simulink model "entropyModel"  (R2024a)
settings: Solver=ode45  StartTime=0.0  StopTime=500  MaxStep=0.1  RelTol=1e-6  AbsTol=1e-6  EnableMultiTasking=on
PreLoadFcn:
  | entropyModelParam;
InitFcn:
  | entropyModelParam;
model workspace (MAT data in the model file):
  cBall = 1000
  cBorder = 1000
  tRegBall = 0.0001
  tRegBorder = 0.0001
undefined symbols (not defined in the file): S1, S10, S2, S3, S4, S5, S6, S7, S8, S9, squareDim, X, Y, Z
libraries: sm_lib x18, nesl_utility x1
settings Model: Creator=lnicolet  LastModifiedBy=lnicolet
settings SolverCC: AutoScaleAbsTol=off  AlgebraicLoopSolver=TrustRegion  MaxZcPerStep=1
settings DataIOCC: LimitDataPoints=on  MaxDataPoints=10000  SaveOutput=off  DSMLogging=off  SaveTime=off  ReturnWorkspaceOutputsName=entropyModelOut
settings OptimizationCC: ReuseModelBlockBuffer=off  LifeSpan=inf
settings DebuggingCC: UnconnectedInputMsg=warning  UnconnectedOutputMsg=warning  UnconnectedLineMsg=warning  AllowSymbolicDim=off  SubsystemReferenceDiagnosticForUnitTest=warning  SFUnexpectedBacktrackingDiag=warning  SFNoUnconditionalDefaultTransitionDiag=warning  SFExecutionAtInitializationDiag=none  ArithmeticOperatorsInVariantConditions=warning
settings ModelReferenceCC: EnableRefExpFcnMdlSchedulingChecks=on
settings SFSimCC: SimUseLocalCustomCode=off  CustomCodeUndefinedFunction=UseInterfaceOnly
settings RTWCC: RTWUseLocalCustomCode=off  GPUComputeCapability=3.5  DLArmComputeVersion=19.05
settings CodeAppCC: StateflowObjectComments=on
settings GRTTargetCC: TargetLangStandard=C89/C90 (ANSI)
settings ConfigComp: CovMetricSettings=dw  CovSaveCumulativeToWorkspaceVar=on  CovSaveSingleToWorkspaceVar=on  CovExternalEMLEnable=off  CovSFcnEnable=off
settings SimscapeCC: SimscapeLogType=all  SimscapeLogSimulationStatistics=on  SimscapeLogLimitData=off  SimscapeLogDataHistory=10000
settings ExplorerConfigSet: InternalSimMechanicsExplorerSettings="<ExplorerConfiguration><canonicalview>default</canonicalview><AnimationSetting><BasePlaybackSpeed>1.0</BasePlaybackSpeed><PlaybackSpeedFactor>8.0</PlaybackSpeedFactor></AnimationSetting><TilePanel><TileInfo><Tiles Columns=\"1\" Count=\"1\" Rows=\"1\"><Column Weight=\"1\"/><Row Weight=\"1\"/><Tile Height=\"1\" Width=\"1\" X=\"0\" Y=\"0\"/></Tiles></TileInfo><SceneInfo><SceneViewer><BGColor><R>0.60000002384185791</R><G>0.60000002384185791</G><B>0.60000002384185791</B></BGColor><Camera><DoPerspective>off</DoPerspective><Position><X>6.2369504360280299</X><Y>-6.23695044572088086</Y><Z>6.23695057144752774</Z></Position><Center><X>-5.10769893583727458e-07</X><Y>5.01077043348848089e-07</Y><Z>-3.75350395915658431e-07</Z></Center><Up><X>-0.408248290463863073</X><Y>0.408248290463863073</Y><Z>0.816496580927726145</Z></Up><ViewLimDist>1</ViewLimDist><YLim>7.04330336570739757</YLim><XLim>9.6408852888040304</XLim></Camera></SceneViewer></SceneInfo></TilePanel><MechEditorPanel><Cameras/><GfxPanelCameraMap/><VideoCreator><PlaybackSpeedRatio>1.0</PlaybackSpeedRatio><FrameRate>30</FrameRate><VideoFormat>Motion JPEG AVI</VideoFormat><FrameSize>auto</FrameSize></VideoCreator></MechEditorPanel></ExplorerConfiguration>"

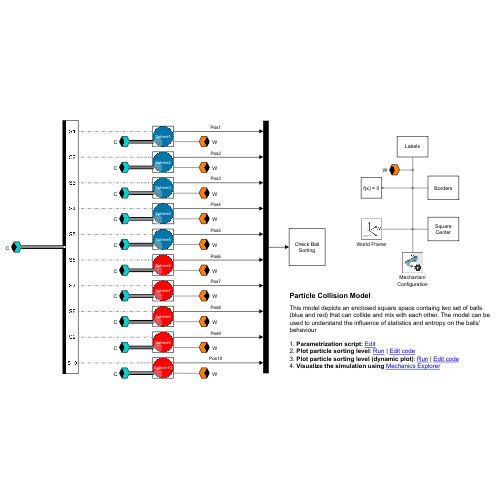
[thumbnail: Simulink's stored preview of the top-level diagram]
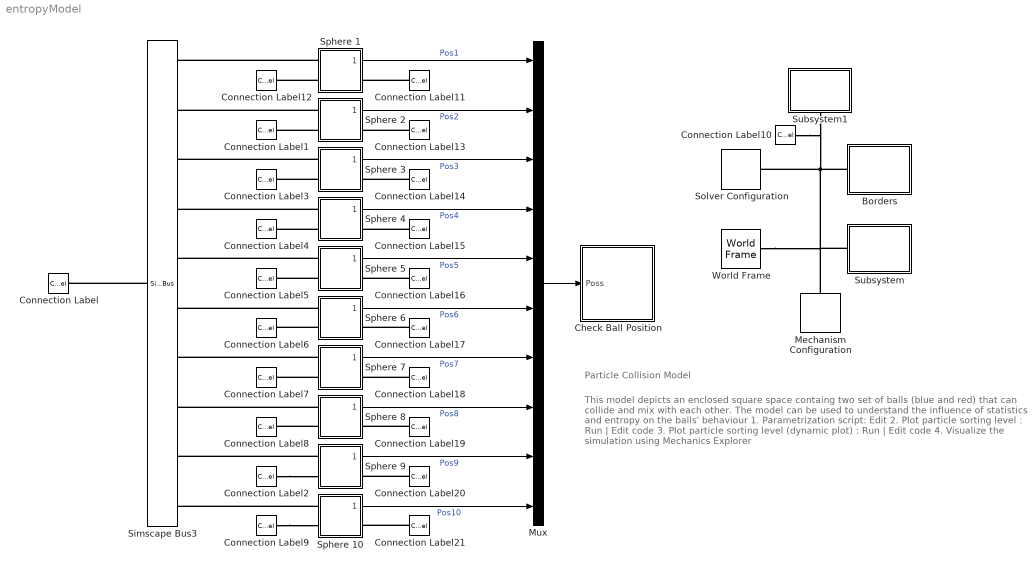
== system entropyModel ==
  note: This model depicts an enclosed square space containg two set of balls (blue and red) that can collide and mix with each other. The model can be used to understand the influence of statistics and entropy on the balls' behaviour
      |
      | 1. Parametrization script: Edit
      | 2. Plot particle sorting level : Run | Edit code
      | 3. Plot particle sorting level (dynamic plot) : Run | Edit code
      | 4. Visualize the simulation using Mechanics Explorer
  note: Particle Collision Model
  Borders : Subsystem
      mask Display: disp('Borders')
  Check Ball Position : Subsystem
      mask Display: disp('Check Ball\nSorting')
  Connection Label{,1..9,12} (11 alike) : ConnectionLabel  Label=C
  Connection Label{10..11,13..21} (11 alike) : ConnectionLabel  Label=W
  Mechanism Configuration : sm_lib/Utilities/Mechanism Configuration  UniformGravity=None  GravityVector=[0 0 -9.80665]  GravityVectorUnits=m/s^2  LinearizationDelta=0.001  JointModeTransitionNonlinearIterations=2
  Mux : Mux  Inputs=10
  Simscape Bus3 : SimscapeBus  HierarchyStrings=S1;S2;S3;S4;S5;S6;S7;S8;S9;S10
  Solver Configuration : nesl_utility/Solver Configuration  PhysicalDomain=network_engine_domain  SubClassName=solver  LeftPortType=input  RightPortType=generic  Tones=[]  Harmonics=[]  SimulateNoise=off  Profile=off  UseLocalSampling=off  EnableSwitchedLinearOptims=on  FrequencyDomain=off  UseCCode=off  RelTol=0.001  AbsTol=1e-06  MinStep=1e-09  ToWorkspace=off  RevertToSquareIcSolve=off  NumHomotopyIterations=100  PhasorMode=off  PhasorModeNumHarmonics=1  ConsistencySolver=NEWTON_XTOL_AFTER_FTOL  IndexReductionMethod=DerivativeReplacement  DoDC=off  ResidualTolerance=1e-09  ConsistencyTolSource=GLOBAL  ConsistencyAbsTol=0.001  ConsistencyRelTol=0.001  ConsistencyTolFactor=0.001  UseLocalSolver=off  LocalSolverChoice=NE_BACKWARD_EULER_ADVANCER  ResolveIndetEquations=on  FunctionEvalNumThread=1  LocalSolverSampleTime=0.001  DoFixedCost=off  MaxNonlinIter=3  MaxModeIter=2  ComputeImpulses=off  ImpulseIterations=2  LinearAlgebra=Sparse  LinearAlgebraNumThread=0  EquationFormulation=NE_TIME_EF  DelaysMemoryBudget=1024  AutomaticFiltering=on  FilteringTimeConstant=0.001  PartitionStorageMethod=AS_NEEDED  PartitionMemoryBudget=1024  PartitionMethod=FAST  MultibodyUseLocalSolver=off  MultibodyLocalSolverChoice=ODE1  MultibodyLocalSolverSampleTime=0.001
  Sphere 1 : Subsystem  ReferencedSubsystem=sphereModel  radius=radiusBall  massBall=massBall  squareDim=squareDim  posMat=posMat  speedMat=speedMat  numBall=1  ballColor=Blue  cBall=cBall  tRegBall=tRegBall  cBorder=cBorder  tRegBorder=tRegBorder
  Sphere 10 : Subsystem  ReferencedSubsystem=sphereModel  radius=radiusBall  massBall=massBall  squareDim=squareDim  posMat=posMat  speedMat=speedMat  numBall=10  ballColor=Red  cBall=cBall  tRegBall=tRegBall  cBorder=cBorder  tRegBorder=tRegBorder
  Sphere 2 : Subsystem  ReferencedSubsystem=sphereModel  radius=radiusBall  massBall=massBall  squareDim=squareDim  posMat=posMat  speedMat=speedMat  numBall=2  ballColor=Blue  cBall=cBall  tRegBall=tRegBall  cBorder=cBorder  tRegBorder=tRegBorder
  Sphere 3 : Subsystem  ReferencedSubsystem=sphereModel  radius=radiusBall  massBall=massBall  squareDim=squareDim  posMat=posMat  speedMat=speedMat  numBall=3  ballColor=Blue  cBall=cBall  tRegBall=tRegBall  cBorder=cBorder  tRegBorder=tRegBorder
  Sphere 4 : Subsystem  ReferencedSubsystem=sphereModel  radius=radiusBall  massBall=massBall  squareDim=squareDim  posMat=posMat  speedMat=speedMat  numBall=4  ballColor=Blue  cBall=cBall  tRegBall=tRegBall  cBorder=cBorder  tRegBorder=tRegBorder
  Sphere 5 : Subsystem  ReferencedSubsystem=sphereModel  radius=radiusBall  massBall=massBall  squareDim=squareDim  posMat=posMat  speedMat=speedMat  numBall=5  ballColor=Blue  cBall=cBall  tRegBall=tRegBall  cBorder=cBorder  tRegBorder=tRegBorder
  Sphere 6 : Subsystem  ReferencedSubsystem=sphereModel  radius=radiusBall  massBall=massBall  squareDim=squareDim  posMat=posMat  speedMat=speedMat  numBall=6  ballColor=Red  cBall=cBall  tRegBall=tRegBall  cBorder=cBorder  tRegBorder=tRegBorder
  Sphere 7 : Subsystem  ReferencedSubsystem=sphereModel  radius=radiusBall  massBall=massBall  squareDim=squareDim  posMat=posMat  speedMat=speedMat  numBall=7  ballColor=Red  cBall=cBall  tRegBall=tRegBall  cBorder=cBorder  tRegBorder=tRegBorder
  Sphere 8 : Subsystem  ReferencedSubsystem=sphereModel  radius=radiusBall  massBall=massBall  squareDim=squareDim  posMat=posMat  speedMat=speedMat  numBall=8  ballColor=Red  cBall=cBall  tRegBall=tRegBall  cBorder=cBorder  tRegBorder=tRegBorder
  Sphere 9 : Subsystem  ReferencedSubsystem=sphereModel  radius=radiusBall  massBall=massBall  squareDim=squareDim  posMat=posMat  speedMat=speedMat  numBall=9  ballColor=Red  cBall=cBall  tRegBall=tRegBall  cBorder=cBorder  tRegBorder=tRegBorder
  Subsystem : Subsystem
      mask Display: disp('Square\nCenter')
  Subsystem1 : Subsystem
      mask Display: disp('Labels')
  World Frame : sm_lib/Frames and Transforms/World Frame
  wires:
  Sphere 8/1 -> Mux/8  "Pos8"
  Sphere 7/1 -> Mux/7  "Pos7"
  Sphere 6/1 -> Mux/6  "Pos6"
  Sphere 5/1 -> Mux/5  "Pos5"
  Sphere 4/1 -> Mux/4  "Pos4"
  Sphere 3/1 -> Mux/3  "Pos3"
  Sphere 2/1 -> Mux/2  "Pos2"
  Sphere 1/1 -> Mux/1  "Pos1"
  Sphere 9/1 -> Mux/9  "Pos9"
  Sphere 10/1 -> Mux/10  "Pos10"
  Mux/1 -> Check Ball Position/1(Poss)
  connections:
  Simscape Bus3/RConn1 -- Connection Label/LConn1
  Sphere 1/LConn2 -- Connection Label12/LConn1
  Sphere 1/LConn1 -- Simscape Bus3/LConn1
  Sphere 2/LConn1 -- Simscape Bus3/LConn2
  Sphere 8/LConn1 -- Simscape Bus3/LConn8
  Sphere 7/LConn1 -- Simscape Bus3/LConn7
  Sphere 6/LConn1 -- Simscape Bus3/LConn6
  Sphere 5/LConn1 -- Simscape Bus3/LConn5
  Sphere 3/LConn1 -- Simscape Bus3/LConn3
  Sphere 4/LConn1 -- Simscape Bus3/LConn4
  Sphere 2/LConn2 -- Connection Label1/LConn1
  Sphere 3/LConn2 -- Connection Label3/LConn1
  Sphere 4/LConn2 -- Connection Label4/LConn1
  Sphere 5/LConn2 -- Connection Label5/LConn1
  Sphere 6/LConn2 -- Connection Label6/LConn1
  Sphere 7/LConn2 -- Connection Label7/LConn1
  Sphere 8/LConn2 -- Connection Label8/LConn1
  Sphere 10/LConn1 -- Simscape Bus3/LConn10
  Sphere 9/LConn1 -- Simscape Bus3/LConn9
  Connection Label2/LConn1 -- Sphere 9/LConn2
  Connection Label9/LConn1 -- Sphere 10/LConn2
  Borders/LConn1 -- Subsystem1/LConn1 -- Connection Label10/LConn1 -- Solver Configuration/RConn1 -- World Frame/RConn1 -- Mechanism Configuration/RConn1 -- Subsystem/RConn1
  Connection Label11/LConn1 -- Sphere 1/RConn1
  Connection Label13/LConn1 -- Sphere 2/RConn1
  Connection Label14/LConn1 -- Sphere 3/RConn1
  Connection Label15/LConn1 -- Sphere 4/RConn1
  Connection Label16/LConn1 -- Sphere 5/RConn1
  Connection Label17/LConn1 -- Sphere 6/RConn1
  Connection Label18/LConn1 -- Sphere 7/RConn1
  Connection Label19/LConn1 -- Sphere 8/RConn1
  Connection Label20/LConn1 -- Sphere 9/RConn1
  Connection Label21/LConn1 -- Sphere 10/RConn1

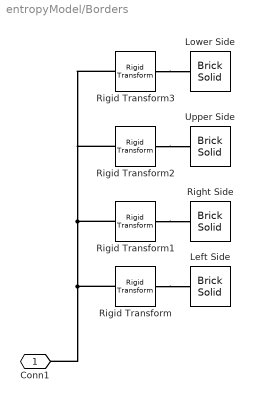
== system entropyModel/Borders ==
  Left Side : sm_lib/Body Elements/Brick Solid  BrickDimensions=[0.05*squareDim, 0.05*squareDim,squareDim]  BrickDimensionsUnits=m  ExportEntireGeometry=off  InertiaType=CalculateFromGeometry  BasedOnType=Density  Density=1000  DensityUnits=kg/m^3  Mass=1  MassUnits=kg  CenterOfMass=[0 0 0]  CenterOfMassUnits=m  MomentsOfInertia=[1 1 1]  MomentsOfInertiaUnits=kg*m^2  ProductsOfInertia=[0 0 0]  ProductsOfInertiaUnits=kg*m^2  GraphicType=FromGeometry  MarkerShape=Sphere  MarkerSize=10  GraphicVisPropType=SimpleVisualProperties  GraphicDiffuseColor=[0,118,168]/255  GraphicOpacity=1.0  GraphicSpecularColor=[0.5 0.5 0.5 1.0]  GraphicAmbientColor=[0.15 0.15 0.15 1.0]  GraphicEmissiveColor=[0.0 0.0 0.0 1.0]  GraphicShininess=75  DoExposeReferenceFrame=on  SerializedFrames=<Frames/>
  Lower Side : sm_lib/Body Elements/Brick Solid  BrickDimensions=[0.05*squareDim, 0.05*squareDim,squareDim*1.1]  BrickDimensionsUnits=m  ExportEntireGeometry=off  InertiaType=CalculateFromGeometry  BasedOnType=Density  Density=1000  DensityUnits=kg/m^3  Mass=1  MassUnits=kg  CenterOfMass=[0 0 0]  CenterOfMassUnits=m  MomentsOfInertia=[1 1 1]  MomentsOfInertiaUnits=kg*m^2  ProductsOfInertia=[0 0 0]  ProductsOfInertiaUnits=kg*m^2  GraphicType=FromGeometry  MarkerShape=Sphere  MarkerSize=10  GraphicVisPropType=SimpleVisualProperties  GraphicDiffuseColor=[0,118,168]/255  GraphicOpacity=1.0  GraphicSpecularColor=[0.5 0.5 0.5 1.0]  GraphicAmbientColor=[0.15 0.15 0.15 1.0]  GraphicEmissiveColor=[0.0 0.0 0.0 1.0]  GraphicShininess=75  DoExposeReferenceFrame=on  SerializedFrames=<Frames/>
  Right Side : sm_lib/Body Elements/Brick Solid  BrickDimensions=[0.05*squareDim, 0.05*squareDim,squareDim]  BrickDimensionsUnits=m  ExportEntireGeometry=off  InertiaType=CalculateFromGeometry  BasedOnType=Density  Density=1000  DensityUnits=kg/m^3  Mass=1  MassUnits=kg  CenterOfMass=[0 0 0]  CenterOfMassUnits=m  MomentsOfInertia=[1 1 1]  MomentsOfInertiaUnits=kg*m^2  ProductsOfInertia=[0 0 0]  ProductsOfInertiaUnits=kg*m^2  GraphicType=FromGeometry  MarkerShape=Sphere  MarkerSize=10  GraphicVisPropType=SimpleVisualProperties  GraphicDiffuseColor=[0,118,168]/255  GraphicOpacity=1.0  GraphicSpecularColor=[0.5 0.5 0.5 1.0]  GraphicAmbientColor=[0.15 0.15 0.15 1.0]  GraphicEmissiveColor=[0.0 0.0 0.0 1.0]  GraphicShininess=75  DoExposeReferenceFrame=on  SerializedFrames=<Frames/>
  Rigid Transform : sm_lib/Frames and Transforms/Rigid Transform  RotationMethod=None  FollAlignAxisA=+X  BaseAlignAxisA=+Y  FollAlignAxisB=+Y  BaseAlignAxisB=+Z  RotationStandardAxis=+Z  RotationAngle=0  RotationAngleUnits=deg  RotationArbitraryAxis=[0 0 1]  RotationSequenceAxes=FollowerAxes  RotationSequence=XYX  RotationSequenceAngles=[0 0 0]  RotationSequenceAnglesUnits=deg  RotationMatrix=[1 0 0;0 1 0;0 0 1]  Quaternion=[1 0 0 0]  TranslationMethod=StandardAxis  TranslationCartesianOffset=[0 0 0]  TranslationCartesianOffsetUnits=m  TranslationStandardAxis=-X  TranslationStandardOffset=squareDim*1.05/2  TranslationStandardOffsetUnits=m  TranslationROffset=0  TranslationROffsetUnits=m  TranslationThetaOffset=0  TranslationThetaOffsetUnits=deg  TranslationZOffset=0  TranslationZOffsetUnits=m
  Rigid Transform1 : sm_lib/Frames and Transforms/Rigid Transform  RotationMethod=None  FollAlignAxisA=+X  BaseAlignAxisA=+Y  FollAlignAxisB=+Y  BaseAlignAxisB=+Z  RotationStandardAxis=+Z  RotationAngle=0  RotationAngleUnits=deg  RotationArbitraryAxis=[0 0 1]  RotationSequenceAxes=FollowerAxes  RotationSequence=XYX  RotationSequenceAngles=[0 0 0]  RotationSequenceAnglesUnits=deg  RotationMatrix=[1 0 0;0 1 0;0 0 1]  Quaternion=[1 0 0 0]  TranslationMethod=StandardAxis  TranslationCartesianOffset=[0 0 0]  TranslationCartesianOffsetUnits=m  TranslationStandardAxis=+X  TranslationStandardOffset=squareDim*1.05/2  TranslationStandardOffsetUnits=m  TranslationROffset=0  TranslationROffsetUnits=m  TranslationThetaOffset=0  TranslationThetaOffsetUnits=deg  TranslationZOffset=0  TranslationZOffsetUnits=m
  Rigid Transform2 : sm_lib/Frames and Transforms/Rigid Transform  RotationMethod=StandardAxis  FollAlignAxisA=+X  BaseAlignAxisA=+Y  FollAlignAxisB=+Y  BaseAlignAxisB=+Z  RotationStandardAxis=+Y  RotationAngle=90  RotationAngleUnits=deg  RotationArbitraryAxis=[0 0 1]  RotationSequenceAxes=FollowerAxes  RotationSequence=XYX  RotationSequenceAngles=[0 0 0]  RotationSequenceAnglesUnits=deg  RotationMatrix=[1 0 0;0 1 0;0 0 1]  Quaternion=[1 0 0 0]  TranslationMethod=StandardAxis  TranslationCartesianOffset=[0 0 0]  TranslationCartesianOffsetUnits=m  TranslationStandardAxis=+Z  TranslationStandardOffset=squareDim*1.05/2  TranslationStandardOffsetUnits=m  TranslationROffset=0  TranslationROffsetUnits=m  TranslationThetaOffset=0  TranslationThetaOffsetUnits=deg  TranslationZOffset=0  TranslationZOffsetUnits=m
  Rigid Transform3 : sm_lib/Frames and Transforms/Rigid Transform  RotationMethod=StandardAxis  FollAlignAxisA=+X  BaseAlignAxisA=+Y  FollAlignAxisB=+Y  BaseAlignAxisB=+Z  RotationStandardAxis=+Y  RotationAngle=90  RotationAngleUnits=deg  RotationArbitraryAxis=[0 0 1]  RotationSequenceAxes=FollowerAxes  RotationSequence=XYX  RotationSequenceAngles=[0 0 0]  RotationSequenceAnglesUnits=deg  RotationMatrix=[1 0 0;0 1 0;0 0 1]  Quaternion=[1 0 0 0]  TranslationMethod=StandardAxis  TranslationCartesianOffset=[0 0 0]  TranslationCartesianOffsetUnits=m  TranslationStandardAxis=+Z  TranslationStandardOffset=-squareDim*1.05/2  TranslationStandardOffsetUnits=m  TranslationROffset=0  TranslationROffsetUnits=m  TranslationThetaOffset=0  TranslationThetaOffsetUnits=deg  TranslationZOffset=0  TranslationZOffsetUnits=m
  Upper Side : sm_lib/Body Elements/Brick Solid  BrickDimensions=[0.05*squareDim, 0.05*squareDim,squareDim*1.1]  BrickDimensionsUnits=m  ExportEntireGeometry=off  InertiaType=CalculateFromGeometry  BasedOnType=Density  Density=1000  DensityUnits=kg/m^3  Mass=1  MassUnits=kg  CenterOfMass=[0 0 0]  CenterOfMassUnits=m  MomentsOfInertia=[1 1 1]  MomentsOfInertiaUnits=kg*m^2  ProductsOfInertia=[0 0 0]  ProductsOfInertiaUnits=kg*m^2  GraphicType=FromGeometry  MarkerShape=Sphere  MarkerSize=10  GraphicVisPropType=SimpleVisualProperties  GraphicDiffuseColor=[0,118,168]/255  GraphicOpacity=1.0  GraphicSpecularColor=[0.5 0.5 0.5 1.0]  GraphicAmbientColor=[0.15 0.15 0.15 1.0]  GraphicEmissiveColor=[0.0 0.0 0.0 1.0]  GraphicShininess=75  DoExposeReferenceFrame=on  SerializedFrames=<Frames/>
  Conn1 : PMIOPort  Side=Left
  connections:
  Rigid Transform3/RConn1 -- Lower Side/RConn1
  Rigid Transform/LConn1 -- Conn1/RConn1 -- Rigid Transform3/LConn1 -- Rigid Transform2/LConn1 -- Rigid Transform1/LConn1
  Rigid Transform1/RConn1 -- Right Side/RConn1
  Rigid Transform/RConn1 -- Left Side/RConn1
  Rigid Transform2/RConn1 -- Upper Side/RConn1

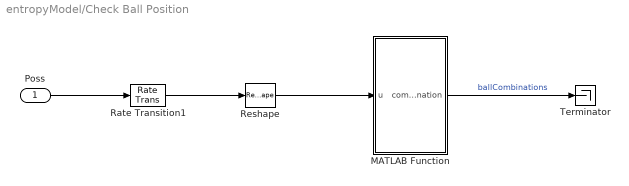
== system entropyModel/Check Ball Position ==
  Poss : Inport
  MATLAB Function : MATLAB Function  TreatAsAtomicUnit=on
  Rate Transition1 : RateTransition  InitialCondition=squareDim  OutPortSampleTime=1
  Reshape : Reshape  OutputDimensionality=Customize  OutputDimensions=[2,10]
  Terminator : Terminator
  wires:
  Poss/1 -> Rate Transition1/1
  Rate Transition1/1 -> Reshape/1
  MATLAB Function/1(combination) -> Terminator/1  "ballCombinations"
  Reshape/1 -> MATLAB Function/1(u)

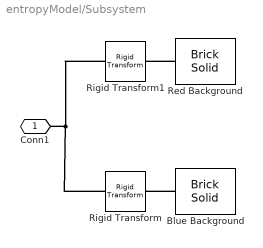
== system entropyModel/Subsystem ==
  Blue Background : sm_lib/Body Elements/Brick Solid  BrickDimensions="[squareDim/2  0.01 squareDim]"  BrickDimensionsUnits=m  ExportEntireGeometry=off  InertiaType=CalculateFromGeometry  BasedOnType=Density  Density=1000  DensityUnits=kg/m^3  Mass=1  MassUnits=kg  CenterOfMass=[0 0 0]  CenterOfMassUnits=m  MomentsOfInertia=[1 1 1]  MomentsOfInertiaUnits=kg*m^2  ProductsOfInertia=[0 0 0]  ProductsOfInertiaUnits=kg*m^2  GraphicType=FromGeometry  MarkerShape=Sphere  MarkerSize=10  GraphicVisPropType=SimpleVisualProperties  GraphicDiffuseColor=[0,0,1]  GraphicOpacity=0.1  GraphicSpecularColor=[0.5 0.5 0.5 1.0]  GraphicAmbientColor=[0.15 0.15 0.15 1.0]  GraphicEmissiveColor=[0.0 0.0 0.0 1.0]  GraphicShininess=75  DoExposeReferenceFrame=on  SerializedFrames=<Frames/>
  Red Background : sm_lib/Body Elements/Brick Solid  BrickDimensions="[squareDim/2  0.01 squareDim]"  BrickDimensionsUnits=m  ExportEntireGeometry=off  InertiaType=CalculateFromGeometry  BasedOnType=Density  Density=1000  DensityUnits=kg/m^3  Mass=1  MassUnits=kg  CenterOfMass=[0 0 0]  CenterOfMassUnits=m  MomentsOfInertia=[1 1 1]  MomentsOfInertiaUnits=kg*m^2  ProductsOfInertia=[0 0 0]  ProductsOfInertiaUnits=kg*m^2  GraphicType=FromGeometry  MarkerShape=Sphere  MarkerSize=10  GraphicVisPropType=SimpleVisualProperties  GraphicDiffuseColor=[1,0,0]  GraphicOpacity=0.1  GraphicSpecularColor=[0.5 0.5 0.5 1.0]  GraphicAmbientColor=[0.15 0.15 0.15 1.0]  GraphicEmissiveColor=[0.0 0.0 0.0 1.0]  GraphicShininess=75  DoExposeReferenceFrame=on  SerializedFrames=<Frames/>
  Rigid Transform : sm_lib/Frames and Transforms/Rigid Transform  RotationMethod=None  FollAlignAxisA=+X  BaseAlignAxisA=+Y  FollAlignAxisB=+Y  BaseAlignAxisB=+Z  RotationStandardAxis=+Z  RotationAngle=0  RotationAngleUnits=deg  RotationArbitraryAxis=[0 0 1]  RotationSequenceAxes=FollowerAxes  RotationSequence=XYX  RotationSequenceAngles=[0 0 0]  RotationSequenceAnglesUnits=deg  RotationMatrix=[1 0 0;0 1 0;0 0 1]  Quaternion=[1 0 0 0]  TranslationMethod=StandardAxis  TranslationCartesianOffset=[0 0 0]  TranslationCartesianOffsetUnits=m  TranslationStandardAxis=+X  TranslationStandardOffset=-squareDim/4  TranslationStandardOffsetUnits=m  TranslationROffset=0  TranslationROffsetUnits=m  TranslationThetaOffset=0  TranslationThetaOffsetUnits=deg  TranslationZOffset=0  TranslationZOffsetUnits=m
  Rigid Transform1 : sm_lib/Frames and Transforms/Rigid Transform  RotationMethod=None  FollAlignAxisA=+X  BaseAlignAxisA=+Y  FollAlignAxisB=+Y  BaseAlignAxisB=+Z  RotationStandardAxis=+Z  RotationAngle=0  RotationAngleUnits=deg  RotationArbitraryAxis=[0 0 1]  RotationSequenceAxes=FollowerAxes  RotationSequence=XYX  RotationSequenceAngles=[0 0 0]  RotationSequenceAnglesUnits=deg  RotationMatrix=[1 0 0;0 1 0;0 0 1]  Quaternion=[1 0 0 0]  TranslationMethod=StandardAxis  TranslationCartesianOffset=[0 0 0]  TranslationCartesianOffsetUnits=m  TranslationStandardAxis=+X  TranslationStandardOffset=squareDim/4  TranslationStandardOffsetUnits=m  TranslationROffset=0  TranslationROffsetUnits=m  TranslationThetaOffset=0  TranslationThetaOffsetUnits=deg  TranslationZOffset=0  TranslationZOffsetUnits=m
  Conn1 : PMIOPort  Side=Right
  connections:
  Conn1/RConn1 -- Rigid Transform1/RConn1 -- Rigid Transform/RConn1
  Blue Background/RConn1 -- Rigid Transform/LConn1
  Red Background/RConn1 -- Rigid Transform1/LConn1

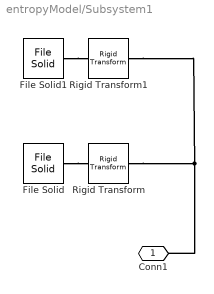
== system entropyModel/Subsystem1 ==
  File Solid : sm_lib/Body Elements/File Solid  ExtGeomFileName=leftLabel.stl  UnitType=Custom  ExtGeomFileUnits=m  StepReaderType=HEX  ExportConvexHullGeometry=off  InertiaType=PointMass  BasedOnType=DensityFromFile  Density=1000  DensityUnits=kg/m^3  Mass=1  MassUnits=kg  CenterOfMass=[0 0 0]  CenterOfMassUnits=m  MomentsOfInertia=[1 1 1]  MomentsOfInertiaUnits=kg*m^2  ProductsOfInertia=[0 0 0]  ProductsOfInertiaUnits=kg*m^2  GraphicType=FromGeometry  MarkerShape=Sphere  MarkerSize=10  GraphicVisPropType=SimpleVisualProperties  GraphicDiffuseColor=[1,0,0]  GraphicOpacity=1  GraphicSpecularColor=[0.5 0.5 0.5 1.0]  GraphicAmbientColor=[0.15 0.15 0.15 1.0]  GraphicEmissiveColor=[0.0 0.0 0.0 1.0]  GraphicShininess=75  DoExposeReferenceFrame=on  SerializedFrames=<Frames/>
  File Solid1 : sm_lib/Body Elements/File Solid  ExtGeomFileName=rightLabel.stl  UnitType=Custom  ExtGeomFileUnits=m  StepReaderType=HEX  ExportConvexHullGeometry=off  InertiaType=PointMass  BasedOnType=DensityFromFile  Density=1000  DensityUnits=kg/m^3  Mass=1  MassUnits=kg  CenterOfMass=[0 0 0]  CenterOfMassUnits=m  MomentsOfInertia=[1 1 1]  MomentsOfInertiaUnits=kg*m^2  ProductsOfInertia=[0 0 0]  ProductsOfInertiaUnits=kg*m^2  GraphicType=FromGeometry  MarkerShape=Sphere  MarkerSize=10  GraphicVisPropType=SimpleVisualProperties  GraphicDiffuseColor=[0,0,1]  GraphicOpacity=1  GraphicSpecularColor=[0.5 0.5 0.5 1.0]  GraphicAmbientColor=[0.15 0.15 0.15 1.0]  GraphicEmissiveColor=[0.0 0.0 0.0 1.0]  GraphicShininess=75  DoExposeReferenceFrame=on  SerializedFrames=<Frames/>
  Rigid Transform : sm_lib/Frames and Transforms/Rigid Transform  RotationMethod=StandardAxis  FollAlignAxisA=+X  BaseAlignAxisA=+Y  FollAlignAxisB=+Y  BaseAlignAxisB=+Z  RotationStandardAxis=-X  RotationAngle=90  RotationAngleUnits=deg  RotationArbitraryAxis=[0 0 1]  RotationSequenceAxes=FollowerAxes  RotationSequence=XYX  RotationSequenceAngles=[0 0 0]  RotationSequenceAnglesUnits=deg  RotationMatrix=[1 0 0;0 1 0;0 0 1]  Quaternion=[1 0 0 0]  TranslationMethod=Cartesian  TranslationCartesianOffset=[1.4303+squareDim/4 0.2793 0]  TranslationCartesianOffsetUnits=m  TranslationStandardAxis=+Z  TranslationStandardOffset=0  TranslationStandardOffsetUnits=m  TranslationROffset=0  TranslationROffsetUnits=m  TranslationThetaOffset=0  TranslationThetaOffsetUnits=deg  TranslationZOffset=0  TranslationZOffsetUnits=m
  Rigid Transform1 : sm_lib/Frames and Transforms/Rigid Transform  RotationMethod=StandardAxis  FollAlignAxisA=+X  BaseAlignAxisA=+Y  FollAlignAxisB=+Y  BaseAlignAxisB=+Z  RotationStandardAxis=-X  RotationAngle=90  RotationAngleUnits=deg  RotationArbitraryAxis=[0 0 1]  RotationSequenceAxes=FollowerAxes  RotationSequence=XYX  RotationSequenceAngles=[0 0 0]  RotationSequenceAnglesUnits=deg  RotationMatrix=[1 0 0;0 1 0;0 0 1]  Quaternion=[1 0 0 0]  TranslationMethod=Cartesian  TranslationCartesianOffset=[1.6793-squareDim/4 0.3466 0]  TranslationCartesianOffsetUnits=m  TranslationStandardAxis=+Z  TranslationStandardOffset=0  TranslationStandardOffsetUnits=m  TranslationROffset=0  TranslationROffsetUnits=m  TranslationThetaOffset=0  TranslationThetaOffsetUnits=deg  TranslationZOffset=0  TranslationZOffsetUnits=m
  Conn1 : PMIOPort  Side=Left
  connections:
  Rigid Transform/RConn1 -- Conn1/RConn1 -- Rigid Transform1/RConn1
  File Solid/RConn1 -- Rigid Transform/LConn1
  File Solid1/RConn1 -- Rigid Transform1/LConn1

== matlab function entropyModel/Check Ball Position/MATLAB Function ==
  data: u input; combination output
function combination  = fcn(u)

% Position of all balls:
posBalls = u(1,:);

% Colors of all balls: 
colorBalls = u(2,:);

% If a ball is on the right side and it is blue, 
combination = (posBalls>=0 & colorBalls ==1) | (posBalls<0 & colorBalls==2);
